simulink model "SourceBlocks"  (R2021b)
settings: Solver=VariableStepAuto  StartTime=0.0  StopTime=1e-3  RelTol=1e-3
undefined symbols (not defined in the file): waveform
settings Model: Creator=yxb20126  LastModifiedBy=yxb20126

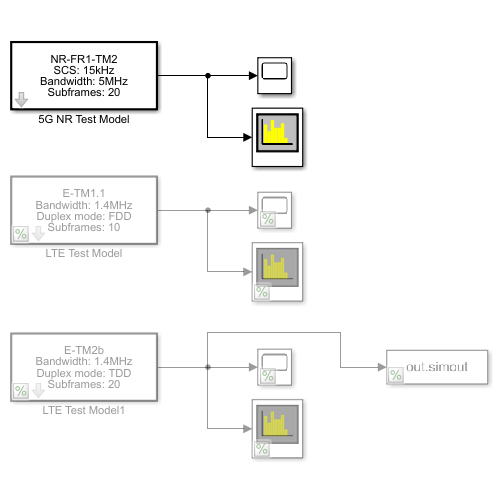
[thumbnail: Simulink's stored preview of the top-level diagram]
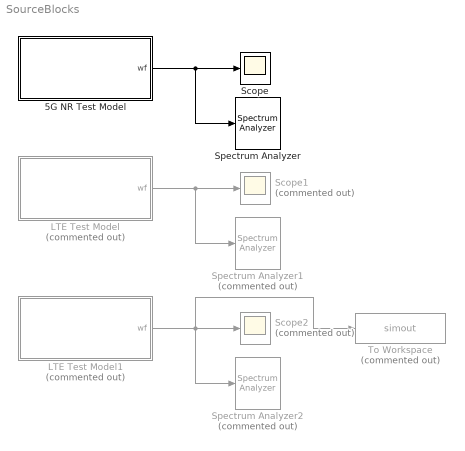
== system SourceBlocks ==
  5G NR Test Model : MATLAB Function  Tag=BlockGeneratedWWGApp  TreatAsAtomicUnit=on  SystemSampleTime=1.3020833333333333957e-07  mask(5G NR Test Model Waveform Generator){waveformLength=153600, nsamps=1, OutputAfterFinalValue=Cyclic repetition}
      mask prompts: waveformLength "Waveform length (samples):"; nsamps "Samples per frame:"; OutputAfterFinalValue "Form output after final data value by:"
      mask help: This block was created using the <a href="matlab:helpview(fullfile(docroot,'toolbox','5g','helptargets.map'),'FiveGWaveformGenerator_app')">5G Waveform Generator</a> app. The block outputs a 5G NR test model waveform corresponding to the MATLAB code available in the Initialization pane of the Mask Editor.<br></br><br>The waveform configuration, sample rate, and length are available in the UserData of the block.</br>
      mask init:
      | %% Generating NR Test Models waveform
      | % NR Test Models configuration
      | cfgDLTM = nrDLCarrierConfig;
      | cfgDLTM.Label = 'NR-FR1-TM2';
      | cfgDLTM.FrequencyRange = 'FR1';
      | cfgDLTM.ChannelBandwidth = 5;
      | cfgDLTM.NCellID = 1;
      | cfgDLTM.NumSubframes = 20;
      | cfgDLTM.WindowingPercent = 0;
      | cfgDLTM.SampleRate = [];
      | cfgDLTM.CarrierFrequency = 0;
      | 
      | %% SCS specific carriers
      | scscarrier = nrSCSCarrierConfig;
      | scscarrier.SubcarrierSpacing = 15;
      | scscarrier.NSizeGrid = 25;
      | scscarrier.NStartGrid = 0;
      | 
      | cfgDLTM.SCSCarriers = {scscarrier};
      | 
      | %% Bandwidth Parts
      | bwp = nrWavegenBWPConfig;
      | bwp.BandwidthPartID = 1;
      | bwp.Label = 'BWP1';
      | bwp.SubcarrierSpacing = 15;
      | bwp.CyclicPrefix = 'normal';
      | bwp.NSizeBWP = 25;
      | bwp.NStartBWP = 0;
      | 
      | cfgDLTM.BandwidthParts = {bwp};
      | 
      | %% Synchronization Signals Burst
      | ssburst = nrWavegenSSBurstConfig;
      | ssburst.BlockPattern = 'Case A';
      | ssburst.TransmittedBlocks = [1 0 0 0];
      | ssburst.Period = 10;
      | ssburst.NCRBSSB = [];
      | ssburst.KSSB = 0;
      | ssburst.DataSource = 'MIB';
      | ssburst.DMRSTypeAPosition = 2;
      | ssburst.CellBarred = false;
      | ssburst.IntraFreqReselection = false;
      | ssburst.PDCCHConfigSIB1 = 0;
      | ssburst.SubcarrierSpacingCommon = 30;
      | ssburst.Enable = false;
      | ssburst.Power = 0;
      | 
      | cfgDLTM.SSBurst = ssburst;
      | 
      | %% CORESET and Search Space Configuration
      | coreset = nrCORESETConfig;
      | coreset.CORESETID = 1;
      | coreset.Label = 'CORESET1';
      | coreset.FrequencyResources = 1;
      | coreset.Duration = 2;
      | coreset.CCEREGMapping = 'noninterleaved';
      | coreset.REGBundleSize = 2;
      | coreset.InterleaverSize = 2;
      | coreset.ShiftIndex = 0;
      | 
      | cfgDLTM.CORESET = {coreset};
      | 
      | % Search Spaces
      | searchspace = nrSearchSpaceConfig;
      | searchspace.SearchSpaceID = 1;
      | searchspace.Label = 'SearchSpace1';
      | searchspace.CORESETID = 1;
      | searchspace.SearchSpaceType = 'common';
      | searchspace.StartSymbolWithinSlot = 0;
      | searchspace.SlotPeriodAndOffset = [1 0];
      | searchspace.Duration = 1;
      | searchspace.NumCandidates = [8 8 0 0 0];
      | 
      | cfgDLTM.SearchSpaces = {searchspace};
      | 
      | %% PDCCH Instances Configuration
      | pdcch = nrWavegenPDCCHConfig;
      | pdcch.Enable = true;
      | pdcch.Label = 'PDCCH1';
      | pdcch.Power = 0;
      | pdcch.BandwidthPartID = 1;
      | pdcch.SearchSpaceID = 1;
      | pdcch.AggregationLevel = 1;
      | pdcch.AllocatedCandidate = 1;
      | pdcch.SlotAllocation = 0:3;
      | pdcch.Period = 5;
      | pdcch.Coding = false;
      | pdcch.DataBlockSize = 20;
      | pdcch.DataSource = 'PN23';
      | pdcch.RNTI = 0;
      | pdcch.DMRSScramblingID = 1;
      | pdcch.DMRSPower = 0;
      | 
      | cfgDLTM.PDCCH = {pdcch};
      | 
      | %% PDSCH Instances Configuration
      | % PDSCH 1
      | pdsch1 = nrWavegenPDSCHConfig;
      | pdsch1.Enable = true;
      | pdsch1.Label = 'PDSCH sequence for lower PRB (3n slots) (Full downlink slots)';
      | pdsch1.Power = 0;
      | pdsch1.BandwidthPartID = 1;
      | pdsch1.Modulation = '64QAM';
      | pdsch1.NumLayers = 1;
      | pdsch1.MappingType = 'A';
      | pdsch1.ReservedCORESET = [];
      | pdsch1.SymbolAllocation = [2 12];
      | pdsch1.SlotAllocation = [0 6];
      | pdsch1.Period = 10;
      | pdsch1.PRBSet = 0;
      | pdsch1.VRBToPRBInterleaving = 0;
      | pdsch1.VRBBundleSize = 2;
      | pdsch1.NID = [];
      | pdsch1.RNTI = 2;
      | pdsch1.Coding = false;
      | pdsch1.TargetCodeRate = 0.4785;
      | pdsch1.TBScaling = 1;
      | pdsch1.XOverhead = 0;
      | pdsch1.RVSequence = 0;
      | pdsch1.DataSource = 'PN23';
      | pdsch1.DMRSPower = 0;
      | pdsch1.EnablePTRS = false;
      | pdsch1.PTRSPower = 0;
      | 
      | % PDSCH Reserved PRB
      | pdsch1ReservedPRB = nrPDSCHReservedConfig;
      | pdsch1ReservedPRB.PRBSet = 0:2;
      | pdsch1ReservedPRB.SymbolSet = [0 1];
      | pdsch1ReservedPRB.Period = 1;
      | 
      | pdsch1.ReservedPRB = {pdsch1ReservedPRB};
      | 
      | % PDSCH DM-RS
      | pdsch1DMRS = nrPDSCHDMRSConfig;
      | pdsch1DMRS.DMRSConfigurationType = 1;
      | pdsch1DMRS.DMRSReferencePoint = 'CRB0';
      | pdsch1DMRS.DMRSTypeAPosition = 2;
      | pdsch1DMRS.DMRSAdditionalPosition = 1;
      | pdsch1DMRS.DMRSLength = 1;
      | pdsch1DMRS.CustomSymbolSet = [];
      | pdsch1DMRS.DMRSPortSet = [];
      | pdsch1DMRS.NIDNSCID = [];
      | pdsch1DMRS.NSCID = 0;
      | pdsch1DMRS.NumCDMGroupsWithoutData = 1;
      | 
      | pdsch1.DMRS = pdsch1DMRS;
      | 
      | % PDSCH PT-RS
      | pdsch1PTRS = nrPDSCHPTRSConfig;
      | pdsch1PTRS.TimeDensity = 4;
      | pdsch1PTRS.FrequencyDensity = 2;
      | pdsch1PTRS.REOffset = '00';
      | pdsch1PTRS.PTRSPortSet = [];
      | 
      | pdsch1.PTRS = pdsch1PTRS;
      | 
      | % PDSCH 2
      | pdsch2 = nrWavegenPDSCHConfig;
      | pdsch2.Enable = true;
      | pdsch2.Label = 'PDSCH sequence for middle PRB (3n+1 slots) (Full downlink slots)';
      | pdsch2.Power = 0;
      | pdsch2.BandwidthPartID = 1;
      | pdsch2.Modulation = '64QAM';
      | pdsch2.NumLayers = 1;
      | pdsch2.MappingType = 'A';
      | pdsch2.ReservedCORESET = [];
      | pdsch2.SymbolAllocation = [2 12];
      | pdsch2.SlotAllocation = [1 7];
      | pdsch2.Period = 10;
      | pdsch2.PRBSet = 12;
      | pdsch2.VRBToPRBInterleaving = 0;
      | pdsch2.VRBBundleSize = 2;
      | pdsch2.NID = [];
      | pdsch2.RNTI = 2;
      | pdsch2.Coding = false;
      | pdsch2.TargetCodeRate = 0.4785;
      | pdsch2.TBScaling = 1;
      | pdsch2.XOverhead = 0;
      | pdsch2.RVSequence = 0;
      | pdsch2.DataSource = 'PN23';
      | pdsch2.DMRSPower = 0;
      | pdsch2.EnablePTRS = false;
      | pdsch2.PTRSPower = 0;
      | 
      | pdschreserved = nrPDSCHReservedConfig;
      | pdschreserved.PRBSet = 0:2;
      | pdschreserved.SymbolSet = [0 1];
      | pdschreserved.Period = 1;
      | 
      | pdsch2.ReservedPRB = {pdschreserved};
      | 
      | pdschdmrs = nrPDSCHDMRSConfig;
      | pdschdmrs.DMRSConfigurationType = 1;
      | pdschdmrs.DMRSReferencePoint = 'CRB0';
      | pdschdmrs.DMRSTypeAPosition = 2;
      | pdschdmrs.DMRSAdditionalPosition = 1;
      | pdschdmrs.DMRSLength = 1;
      | pdschdmrs.CustomSymbolSet = [];
      | pdschdmrs.DMRSPortSet = [];
      | pdschdmrs.NIDNSCID = [];
      | pdschdmrs.NSCID = 0;
      | pdschdmrs.NumCDMGroupsWithoutData = 1;
      | 
      | pdsch2.DMRS = pdschdmrs;
      | 
      | pdschptrs = nrPDSCHPTRSConfig;
      | pdschptrs.TimeDensity = 4;
      | pdschptrs.FrequencyDensity = 2;
      | pdschptrs.REOffset = '00';
      | pdschptrs.PTRSPortSet = [];
      | 
      | pdsch2.PTRS = pdschptrs;
      | 
      | % PDSCH 3
      | pdsch3 = nrWavegenPDSCHConfig;
      | pdsch3.Enable = true;
      | pdsch3.Label = 'PDSCH sequence for upper PRB (3n+2 slots) (Full downlink slots)';
      | pdsch3.Power = 0;
      | pdsch3.BandwidthPartID = 1;
      | pdsch3.Modulation = '64QAM';
      | pdsch3.NumLayers = 1;
      | pdsch3.MappingType = 'A';
      | pdsch3.ReservedCORESET = [];
      | pdsch3.SymbolAllocation = [2 12];
      | pdsch3.SlotAllocation = [2 5];
      | pdsch3.Period = 10;
      | pdsch3.PRBSet = 24;
      | pdsch3.VRBToPRBInterleaving = 0;
      | pdsch3.VRBBundleSize = 2;
      | pdsch3.NID = [];
      | pdsch3.RNTI = 2;
      | pdsch3.Coding = false;
      | pdsch3.TargetCodeRate = 0.4785;
      | pdsch3.TBScaling = 1;
      | pdsch3.XOverhead = 0;
      | pdsch3.RVSequence = 0;
      | pdsch3.DataSource = 'PN23';
      | pdsch3.DMRSPower = 0;
      | pdsch3.EnablePTRS = false;
      | pdsch3.PTRSPower = 0;
      | 
      | pdschreserved = nrPDSCHReservedConfig;
      | pdschreserved.PRBSet = 0:2;
      | pdschreserved.SymbolSet = [0 1];
      | pdschreserved.Period = 1;
      | 
      | pdsch3.ReservedPRB = {pdschreserved};
      | 
      | pdschdmrs = nrPDSCHDMRSConfig;
      | pdschdmrs.DMRSConfigurationType = 1;
      | pdschdmrs.DMRSReferencePoint = 'CRB0';
      | pdschdmrs.DMRSTypeAPosition = 2;
      | pdschdmrs.DMRSAdditionalPosition = 1;
      | pdschdmrs.DMRSLength = 1;
      | pdschdmrs.CustomSymbolSet = [];
      | pdschdmrs.DMRSPortSet = [];
      | pdschdmrs.NIDNSCID = [];
      | pdschdmrs.NSCID = 0;
      | pdschdmrs.NumCDMGroupsWithoutData = 1;
      | 
      | pdsch3.DMRS = pdschdmrs;
      | 
      | pdschptrs = nrPDSCHPTRSConfig;
      | pdschptrs.TimeDensity = 4;
      | pdschptrs.FrequencyDensity = 2;
      | pdschptrs.REOffset = '00';
      | pdschptrs.PTRSPortSet = [];
      | 
      | pdsch3.PTRS = pdschptrs;
      | 
      | % PDSCH 4
      | pdsch4 = nrWavegenPDSCHConfig;
      | pdsch4.Enable = true;
      | pdsch4.Label = 'PDSCH sequence for lower PRB (3n slots) (Partial downlink slots)';
      | pdsch4.Power = 0;
      | pdsch4.BandwidthPartID = 1;
      | pdsch4.Modulation = '64QAM';
      | pdsch4.NumLayers = 1;
      | pdsch4.MappingType = 'A';
      | pdsch4.ReservedCORESET = [];
      | pdsch4.SymbolAllocation = [2 8];
      | pdsch4.SlotAllocation = 3;
      | pdsch4.Period = 10;
      | pdsch4.PRBSet = 0;
      | pdsch4.VRBToPRBInterleaving = 0;
      | pdsch4.VRBBundleSize = 2;
      | pdsch4.NID = [];
      | pdsch4.RNTI = 2;
      | pdsch4.Coding = false;
      | pdsch4.TargetCodeRate = 0.4785;
      | pdsch4.TBScaling = 1;
      | pdsch4.XOverhead = 0;
      | pdsch4.RVSequence = 0;
      | pdsch4.DataSource = 'PN23';
      | pdsch4.DMRSPower = 0;
      | pdsch4.EnablePTRS = false;
      | pdsch4.PTRSPower = 0;
      | 
      | pdschreserved = nrPDSCHReservedConfig;
      | pdschreserved.PRBSet = 0:2;
      | pdschreserved.SymbolSet = [0 1];
      | pdschreserved.Period = 1;
      | 
      | pdsch4.ReservedPRB = {pdschreserved};
      | 
      | pdschdmrs = nrPDSCHDMRSConfig;
      | pdschdmrs.DMRSConfigurationType = 1;
      | pdschdmrs.DMRSReferencePoint = 'CRB0';
      | pdschdmrs.DMRSTypeAPosition = 2;
      | pdschdmrs.DMRSAdditionalPosition = 1;
      | pdschdmrs.DMRSLength = 1;
      | pdschdmrs.CustomSymbolSet = [];
      | pdschdmrs.DMRSPortSet = [];
      | pdschdmrs.NIDNSCID = [];
      | pdschdmrs.NSCID = 0;
      | pdschdmrs.NumCDMGroupsWithoutData = 1;
      | 
      | pdsch4.DMRS = pdschdmrs;
      | 
      | pdschptrs = nrPDSCHPTRSConfig;
      | pdschptrs.TimeDensity = 4;
      | pdschptrs.FrequencyDensity = 2;
      | pdschptrs.REOffset = '00';
      | pdschptrs.PTRSPortSet = [];
      | 
      | pdsch4.PTRS = pdschptrs;
      | 
      | % PDSCH 5
      | pdsch5 = nrWavegenPDSCHConfig;
      | pdsch5.Enable = true;
      | pdsch5.Label = 'PDSCH sequence for middle PRB (3n+1 slots) (Partial downlink slots)';
      | pdsch5.Power = 0;
      | pdsch5.BandwidthPartID = 1;
      | pdsch5.Modulation = '64QAM';
      | pdsch5.NumLayers = 1;
      | pdsch5.MappingType = 'A';
      | pdsch5.ReservedCORESET = [];
      | pdsch5.SymbolAllocation = [2 8];
      | pdsch5.SlotAllocation = zeros(1,0);
      | pdsch5.Period = 10;
      | pdsch5.PRBSet = 12;
      | pdsch5.VRBToPRBInterleaving = 0;
      | pdsch5.VRBBundleSize = 2;
      | pdsch5.NID = [];
      | pdsch5.RNTI = 2;
      | pdsch5.Coding = false;
      | pdsch5.TargetCodeRate = 0.4785;
      | pdsch5.TBScaling = 1;
      | pdsch5.XOverhead = 0;
      | pdsch5.RVSequence = 0;
      | pdsch5.DataSource = 'PN23';
      | pdsch5.DMRSPower = 0;
      | pdsch5.EnablePTRS = false;
      | pdsch5.PTRSPower = 0;
      | 
      | pdschreserved = nrPDSCHReservedConfig;
      | pdschreserved.PRBSet = 0:2;
      | pdschreserved.SymbolSet = [0 1];
      | pdschreserved.Period = 1;
      | 
      | pdsch5.ReservedPRB = {pdschreserved};
      | 
      | pdschdmrs = nrPDSCHDMRSConfig;
      | pdschdmrs.DMRSConfigurationType = 1;
      | pdschdmrs.DMRSReferencePoint = 'CRB0';
      | pdschdmrs.DMRSTypeAPosition = 2;
      | pdschdmrs.DMRSAdditionalPosition = 1;
      | pdschdmrs.DMRSLength = 1;
      | pdschdmrs.CustomSymbolSet = [];
      | pdschdmrs.DMRSPortSet = [];
      | pdschdmrs.NIDNSCID = [];
      | pdschdmrs.NSCID = 0;
      | pdschdmrs.NumCDMGroupsWithoutData = 1;
      | 
      | pdsch5.DMRS = pdschdmrs;
      | 
      | pdschptrs = nrPDSCHPTRSConfig;
      | pdschptrs.TimeDensity = 4;
      | pdschptrs.FrequencyDensity = 2;
      | pdschptrs.REOffset = '00';
      | pdschptrs.PTRSPortSet = [];
      | 
      | pdsch5.PTRS = pdschptrs;
      | 
      | % PDSCH 6
      | pdsch6 = nrWavegenPDSCHConfig;
      | pdsch6.Enable = true;
      | pdsch6.Label = 'PDSCH sequence for upper PRB (3n+2 slots) (Partial downlink slots)';
      | pdsch6.Power = 0;
      | pdsch6.BandwidthPartID = 1;
      | pdsch6.Modulation = '64QAM';
      | pdsch6.NumLayers = 1;
      | pdsch6.MappingType = 'A';
      | pdsch6.ReservedCORESET = [];
      | pdsch6.SymbolAllocation = [2 8];
      | pdsch6.SlotAllocation = 8;
      | pdsch6.Period = 10;
      | pdsch6.PRBSet = 24;
      | pdsch6.VRBToPRBInterleaving = 0;
      | pdsch6.VRBBundleSize = 2;
      | pdsch6.NID = [];
      | pdsch6.RNTI = 2;
      | pdsch6.Coding = false;
      | pdsch6.TargetCodeRate = 0.4785;
      | pdsch6.TBScaling = 1;
      | pdsch6.XOverhead = 0;
      | pdsch6.RVSequence = 0;
      | pdsch6.DataSource = 'PN23';
      | pdsch6.DMRSPower = 0;
      | pdsch6.EnablePTRS = false;
      | pdsch6.PTRSPower = 0;
      | 
      | pdschreserved = nrPDSCHReservedConfig;
      | pdschreserved.PRBSet = 0:2;
      | pdschreserved.SymbolSet = [0 1];
      | pdschreserved.Period = 1;
      | 
      | pdsch6.ReservedPRB = {pdschreserved};
      | 
      | pdschdmrs = nrPDSCHDMRSConfig;
      | pdschdmrs.DMRSConfigurationType = 1;
      | pdschdmrs.DMRSReferencePoint = 'CRB0';
      | pdschdmrs.DMRSTypeAPosition = 2;
      | pdschdmrs.DMRSAdditionalPosition = 1;
      | pdschdmrs.DMRSLength = 1;
      | pdschdmrs.CustomSymbolSet = [];
      | pdschdmrs.DMRSPortSet = [];
      | pdschdmrs.NIDNSCID = [];
      | pdschdmrs.NSCID = 0;
      | pdschdmrs.NumCDMGroupsWithoutData = 1;
      | 
      | pdsch6.DMRS = pdschdmrs;
      | 
      | pdschptrs = nrPDSCHPTRSConfig;
      | pdschptrs.TimeDensity = 4;
      | pdschptrs.FrequencyDensity = 2;
      | pdschptrs.REOffset = '00';
      | pdschptrs.PTRSPortSet = [];
      | 
      | pdsch6.PTRS = pdschptrs;
      | 
      | cfgDLTM.PDSCH = {pdsch1,pdsch2,pdsch3,pdsch4,pdsch5,pdsch6};
      | 
      | %% CSI-RS Instances Configuration
      | csirs = nrWavegenCSIRSConfig;
      | csirs.Enable = false;
      | csirs.Label = 'CSIRS1';
      | csirs.Power = 0;
      | csirs.BandwidthPartID = 1;
      | csirs.CSIRSType = {'nzp'};
      | csirs.CSIRSPeriod = 'on';
      | csirs.RowNumber = 1;
      | csirs.Density = {'three'};
      | csirs.SymbolLocations = {0};
      | csirs.SubcarrierLocations = {0};
      | csirs.NumRB = 25;
      | csirs.RBOffset = 0;
      | csirs.NID = 1;
      | 
      | cfgDLTM.CSIRS = {csirs};
      | 
      | % Generation
      | [waveform,info] = nrWaveformGenerator(cfgDLTM);
      | 
      | Fs = info.ResourceGrids(1).Info.SampleRate; 								 % Specify the sample rate of the waveform in Hz
      | 
      | % Get current block
      | thisBlock = gcb;
      | 
      | % Evaluate OutputAfterFinalValue to logical type for MFB function
      | OutputAfterFinalValue = strcmp(get_param(thisBlock,'OutputAfterFinalValue'),'Cyclic repetition');
      | 
      | % Set info parameters
      | set_param(thisBlock,'waveformLength',num2str(length(waveform)));
      | maskHandle = Simulink.Mask.get(thisBlock);
      | textFsDialog = maskHandle.getDialogControl('textFs');
      | textFsDialog.Prompt = ['Waveform sample rate (Fs): ' num2str(Fs*1e-6,'%.9g') ' MHz'];
      | textWfLengthDialog = maskHandle.getDialogControl('textWFLength');
      | textWfLengthDialog.Prompt = ['Waveform length: ' num2str(length(waveform)) ' samples'];
      | 
      | % Set sample time of the block
      | set_param(thisBlock, 'SystemSampleTime', num2str(nsamps/Fs,'%.20g'));
      | 
      | % Update UserData
      | outVar.WaveformConfig = cfgDLTM;
      | outVar.WaveformLength = length(waveform);
      | outVar.Fs = Fs;
      | set_param(thisBlock, 'UserData', outVar);
  LTE Test Model : MATLAB Function  Tag=BlockGeneratedWWGApp  Commented=on  TreatAsAtomicUnit=on  SystemSampleTime=5.2083333333333335829e-07  mask(LTE Test Model Waveform Generator){waveformLength=19200, nsamps=1, OutputAfterFinalValue=Cyclic repetition}
      mask prompts: waveformLength "Waveform length (samples):"; nsamps "Samples per frame:"; OutputAfterFinalValue "Form output after final data value by:"
      mask help: This block was created using the <a href="matlab:helpview(fullfile(docroot,'toolbox','lte','helptargets.map'),'LTEWaveformGenerator_app')">LTE Waveform Generator</a> app. The block outputs an LTE test model waveform corresponding to the MATLAB code available in the Initialization pane of the Mask Editor.<br></br><br>The waveform configuration, sample rate, and length are available in the UserData of the block.</br>
      mask init:
      | %% Generating LTE Test Models waveform
      | % LTE Test Models configuration
      | cfg = struct('TMN', '1.1', ...
      |     'BW', '1.4MHz', ...
      |     'NCellID', 1, ...
      |     'DuplexMode', 'FDD', ...
      |     'TotSubframes', 10, ...
      |     'Windowing', 0);
      | 
      | cfg = lteTestModel(cfg);
      | 
      | % Generation
      | [waveform, grid, cfg] = lteTestModelTool(cfg);
      | 
      | Fs = cfg.SamplingRate; 								 % Specify the sample rate of the waveform in Hz
      | 
      | % Get current block
      | thisBlock = gcb;
      | 
      | % Evaluate OutputAfterFinalValue to logical type for MFB function
      | OutputAfterFinalValue = strcmp(get_param(thisBlock,'OutputAfterFinalValue'),'Cyclic repetition');
      | 
      | % Set info parameters
      | set_param(thisBlock,'waveformLength',num2str(length(waveform)));
      | maskHandle = Simulink.Mask.get(thisBlock);
      | textFsDialog = maskHandle.getDialogControl('textFs');
      | textFsDialog.Prompt = ['Waveform sample rate (Fs): ' num2str(Fs*1e-6,'%.9g') ' MHz'];
      | textWfLengthDialog = maskHandle.getDialogControl('textWFLength');
      | textWfLengthDialog.Prompt = ['Waveform length: ' num2str(length(waveform)) ' samples'];
      | 
      | % Set sample time of the block
      | set_param(thisBlock, 'SystemSampleTime', num2str(nsamps/Fs,'%.20g'));
      | 
      | % Update UserData
      | outVar.WaveformConfig = cfg;
      | outVar.WaveformLength = length(waveform);
      | outVar.Fs = Fs;
      | set_param(thisBlock, 'UserData', outVar);
  LTE Test Model1 : MATLAB Function  Tag=BlockGeneratedWWGApp  Commented=on  TreatAsAtomicUnit=on  SystemSampleTime=5.2083333333333335829e-07  mask(LTE Test Model Waveform Generator){waveformLength=38400, nsamps=1, OutputAfterFinalValue=Cyclic repetition}
      mask prompts: waveformLength "Waveform length (samples):"; nsamps "Samples per frame:"; OutputAfterFinalValue "Form output after final data value by:"
      mask help: This block was created using the <a href="matlab:helpview(fullfile(docroot,'toolbox','lte','helptargets.map'),'LTEWaveformGenerator_app')">LTE Waveform Generator</a> app. The block outputs an LTE test model waveform corresponding to the MATLAB code available in the Initialization pane of the Mask Editor.<br></br><br>The waveform configuration, sample rate, and length are available in the UserData of the block.</br>
      mask init:
      | %% Generating LTE Test Models waveform
      | % LTE Test Models configuration
      | cfg = struct('TMN', '2b', ...
      |     'BW', '1.4MHz', ...
      |     'NCellID', 1, ...
      |     'DuplexMode', 'TDD', ...
      |     'TotSubframes', 20, ...
      |     'Windowing', 0);
      | 
      | cfg = lteTestModel(cfg);
      | 
      | % Generation
      | [waveform, grid, cfg] = lteTestModelTool(cfg);
      | 
      | Fs = cfg.SamplingRate; 								 % Specify the sample rate of the waveform in Hz
      | 
      | % Get current block
      | thisBlock = gcb;
      | 
      | % Evaluate OutputAfterFinalValue to logical type for MFB function
      | OutputAfterFinalValue = strcmp(get_param(thisBlock,'OutputAfterFinalValue'),'Cyclic repetition');
      | 
      | % Set info parameters
      | set_param(thisBlock,'waveformLength',num2str(length(waveform)));
      | maskHandle = Simulink.Mask.get(thisBlock);
      | textFsDialog = maskHandle.getDialogControl('textFs');
      | textFsDialog.Prompt = ['Waveform sample rate (Fs): ' num2str(Fs*1e-6,'%.9g') ' MHz'];
      | textWfLengthDialog = maskHandle.getDialogControl('textWFLength');
      | textWfLengthDialog.Prompt = ['Waveform length: ' num2str(length(waveform)) ' samples'];
      | 
      | % Set sample time of the block
      | set_param(thisBlock, 'SystemSampleTime', num2str(nsamps/Fs,'%.20g'));
      | 
      | % Update UserData
      | outVar.WaveformConfig = cfg;
      | outVar.WaveformLength = length(waveform);
      | outVar.Fs = Fs;
      | set_param(thisBlock, 'UserData', outVar);
  Scope : Scope
  Scope1 : Scope  Commented=on
  Scope2 : Scope  Commented=on
  Spectrum Analyzer : SpectrumAnalyzer
  Spectrum Analyzer1 : SpectrumAnalyzer  Commented=on
  Spectrum Analyzer2 : SpectrumAnalyzer  Commented=on
  To Workspace : ToWorkspace  Commented=on  VariableName=simout  SaveFormat=Timeseries  SampleTime=-1
      settings: Save2DSignal=2-D array (concatenate along first dimension)
  wires:
  5G NR Test Model/1(wf) -> Spectrum Analyzer/1, Scope/1
  LTE Test Model/1(wf) -> Spectrum Analyzer1/1, Scope1/1
  LTE Test Model1/1(wf) -> Spectrum Analyzer2/1, To Workspace/1, Scope2/1

== matlab function SourceBlocks/5G NR Test Model ==
  data: wf output; waveform parameter; nsamps parameter; OutputAfterFinalValue parameter
function wf = wfGenerator(waveform, nsamps, OutputAfterFinalValue)

% Create persistent variable
persistent src;

% Preallocate output
wf = complex(zeros(nsamps,size(waveform,2)));

if isempty(src)
    % Get action when signal ends
    if OutputAfterFinalValue
        signalEndAction = 'Cyclic repetition';
    else
        signalEndAction = 'Set to zero';
    end
    
    % Initialize persistent dsp.SignalSource to get current frame
    src = dsp.SignalSource(waveform,nsamps,'SignalEndAction',signalEndAction);
end

% Extract current frame
wf(:,:) = src();

end

== matlab function SourceBlocks/LTE Test Model1 ==
  data: wf output; waveform parameter; nsamps parameter; OutputAfterFinalValue parameter
function wf = wfGenerator(waveform, nsamps, OutputAfterFinalValue)

% Create persistent variable
persistent src;

% Preallocate output
wf = complex(zeros(nsamps,size(waveform,2)));

if isempty(src)
    % Get action when signal ends
    if OutputAfterFinalValue
        signalEndAction = 'Cyclic repetition';
    else
        signalEndAction = 'Set to zero';
    end
    
    % Initialize persistent dsp.SignalSource to get current frame
    src = dsp.SignalSource(waveform,nsamps,'SignalEndAction',signalEndAction);
end

% Extract current frame
wf(:,:) = src();

end

== matlab function SourceBlocks/LTE Test Model ==
  data: wf output; waveform parameter; nsamps parameter; OutputAfterFinalValue parameter
function wf = wfGenerator(waveform, nsamps, OutputAfterFinalValue)

% Create persistent variable
persistent src;

% Preallocate output
wf = complex(zeros(nsamps,size(waveform,2)));

if isempty(src)
    % Get action when signal ends
    if OutputAfterFinalValue
        signalEndAction = 'Cyclic repetition';
    else
        signalEndAction = 'Set to zero';
    end
    
    % Initialize persistent dsp.SignalSource to get current frame
    src = dsp.SignalSource(waveform,nsamps,'SignalEndAction',signalEndAction);
end

% Extract current frame
wf(:,:) = src();

end
